simulink model "oving2d"  (R2020b)
settings: Solver=VariableStepAuto  StartTime=0.0  StopTime=stop_T  MaxStep=max_dt  RelTol=1e-3
undefined symbols (not defined in the file): K, l, T, y_0
settings Model: Creator=crezl  LastModifiedBy=crezl

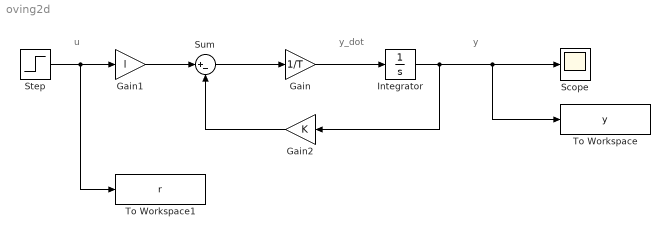
== system oving2d ==
  note: u
  note: y
  note: y_dot
  Gain : Gain  Gain=1/T
  Gain1 : Gain  Gain=l
  Gain2 : Gain  Gain=K
  Integrator : Integrator  InitialCondition=y_0
  Scope : Scope
  Step : Step  Time=0  After=u  SampleTime=0
  Sum : Sum  Inputs=|+-
  To Workspace : ToWorkspace  VariableName=y  SaveFormat=Timeseries  SampleTime=-1
  To Workspace1 : ToWorkspace  VariableName=r  SaveFormat=Timeseries  SampleTime=-1
  wires:
  Gain/1 -> Integrator/1
  Gain1/1 -> Sum/1
  Step/1 -> To Workspace1/1, Gain1/1
  Sum/1 -> Gain/1
  Gain2/1 -> Sum/2
  Integrator/1 -> To Workspace/1, Scope/1, Gain2/1
